simulink model "model1"  (R2016a)
settings: Solver=VariableStepAuto  StartTime=0.0  StopTime=10.0  RelTol=1e-3
settings Model: Creator=malikeh  LastModifiedBy=malikeh

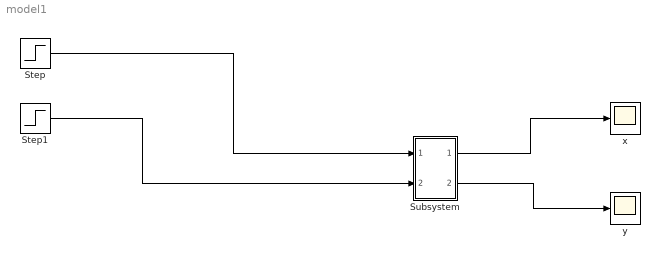
== system model1 ==
  Step : Step  SampleTime=0
  Step1 : Step  SampleTime=0
  Subsystem : Subsystem
  x : Scope
  y : Scope
  wires:
  Step/1 -> Subsystem/1(In1)
  Step1/1 -> Subsystem/2(In2)
  Subsystem/1(Out1) -> x/1
  Subsystem/2(Out2) -> y/1

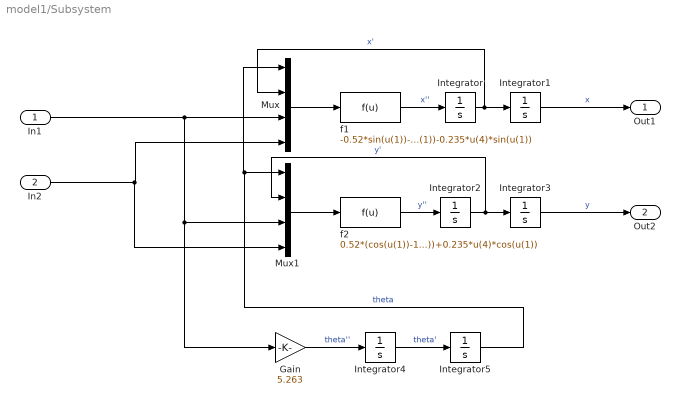
== system model1/Subsystem ==
  In1 : Inport
  In2 : Inport  Port=2
  Gain : Gain  Gain=5.263
  Integrator{,1..5} (6 alike) : Integrator
  Mux : Mux
  Mux1 : Mux
  f1 : Fcn  Expr=-0.52*sin(u(1))-0.0235*u(2)+0.235*u(3)*cos(u(1))-0.235*u(4)*sin(u(1))
  f2 : Fcn  Expr=0.52*(cos(u(1))-1)-0.0235*u(2)+0.235*u(3)*sin(u(1))+0.235*u(4)*cos(u(1))
  Out1 : Outport
  Out2 : Outport  Port=2
  wires:
  Gain/1 -> Integrator4/1  "theta''"
  Integrator5/1 -> Mux1/1, Mux/1  "theta"
  Mux1/1 -> f2/1
  In1/1 -> Gain/1, Mux1/3, Mux/3
  In2/1 -> Mux1/4, Mux/4
  Integrator2/1 -> Integrator3/1, Mux1/2  "y'"
  Integrator1/1 -> Out1/1  "x"
  f2/1 -> Integrator2/1  "y''"
  Integrator3/1 -> Out2/1  "y"
  Integrator/1 -> Integrator1/1, Mux/2  "x'"
  f1/1 -> Integrator/1  "x''"
  Mux/1 -> f1/1
  Integrator4/1 -> Integrator5/1  "theta'"
